simulink subsystem "CompleteController"  (R2022b)
settings: Solver=VariableStepAuto  StartTime=0.0  StopTime=10.0  RelTol=1e-3
settings Model: Creator=Sahil Gaurkar  LastModifiedBy=Sahil Gaurkar

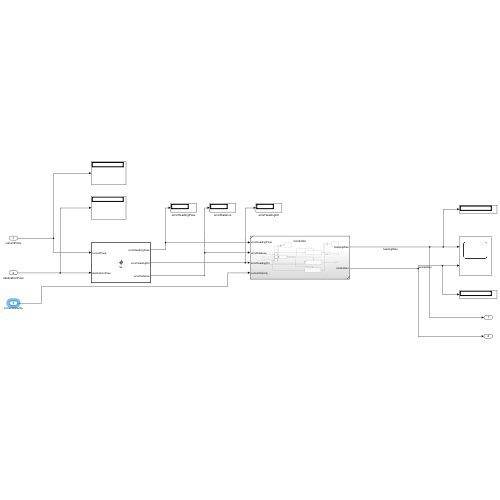
[thumbnail: Simulink's stored preview of the top-level diagram]
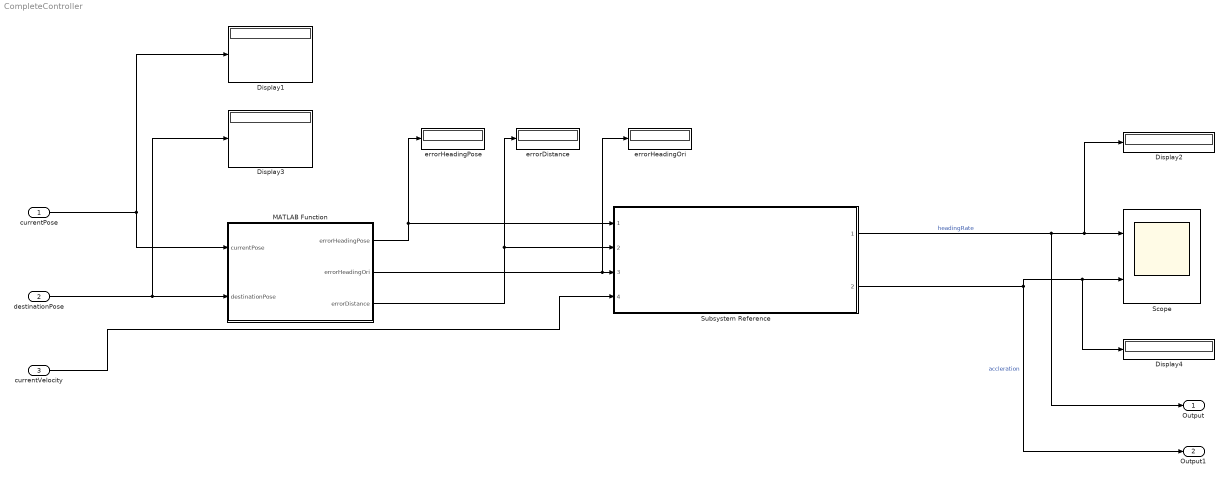
== system CompleteController ==
  currentPose : Inport
  destinationPose : Inport  Port=2
  currentVelocity : Inport  Port=3
  Display{1..4} (4 alike) : Display
  MATLAB Function : MATLAB Function  TreatAsAtomicUnit=on
  Scope : Scope  NumInputPorts=2
  Subsystem Reference : Subsystem  ReferencedSubsystem=Controller
  errorDistance : Display
  errorHeadingOri : Display
  errorHeadingPose : Display
  Output : Outport
  Output1 : Outport  Port=2
  wires:
  currentPose/1 -> MATLAB Function/1(currentPose), Display1/1
  MATLAB Function/3(errorDistance) -> errorDistance/1, Subsystem Reference/2
  destinationPose/1 -> Display3/1, MATLAB Function/2(destinationPose)
  MATLAB Function/2(errorHeadingOri) -> errorHeadingOri/1, Subsystem Reference/3
  Subsystem Reference/2 -> Output1/1, Display4/1, Scope/2  "accleration"
  MATLAB Function/1(errorHeadingPose) -> errorHeadingPose/1, Subsystem Reference/1
  Subsystem Reference/1 -> Output/1, Display2/1, Scope/1  "headingRate"
  currentVelocity/1 -> Subsystem Reference/4

== matlab function CompleteController/MATLAB Function ==
  data: currentPose input; errorHeadingPose output; errorHeadingOri output; destinationPose input; errorDistance output
function [errorHeadingPose, errorHeadingOri, errorDistance] = fcn(currentPose, destinationPose)


errorDistance = sqrt( (destinationPose(1)-currentPose(1))^2 + (destinationPose(2)-currentPose(2))^2 );
errorHeadingPose = atan2d(destinationPose(2) - currentPose(2), destinationPose(1) - currentPose(1)) - currentPose(3);
%errorHeadingPose = round(errorHeadingPose, 3);
%errorHeadingOri = destinationPose(3) - currentPose(3);


if errorHeadingPose > 0.00001
    errorHeadingPose = atan2d(destinationPose(2) - currentPose(2), destinationPose(1) - currentPose(1)) - currentPose(3);
    errorHeadingOri = 0;
    errorDistance = 0;
elseif errorDistance > 10
    errorDistance = sqrt( (destinationPose(1)-currentPose(1))^2 + (destinationPose(2)-currentPose(2))^2 );
    errorHeadingOri = 0;
    errorHeadingPose = 0;
else
    errorHeadingOri = destinationPose(3) - currentPose(3);
    errorHeadingPose = 0;
    errorDistance = 0;
end




end
